simulink model "servoDirection"  (R2019a)
settings: Solver=VariableStepAuto  StartTime=0.0  StopTime=10.0  RelTol=1e-3
undefined symbols (not defined in the file or in its folder): DiscIntNeverNeededParam
libraries: embdlinuxlib x2, raspberrypilib x1
settings Model: Creator=wojna  LastModifiedBy=wojna

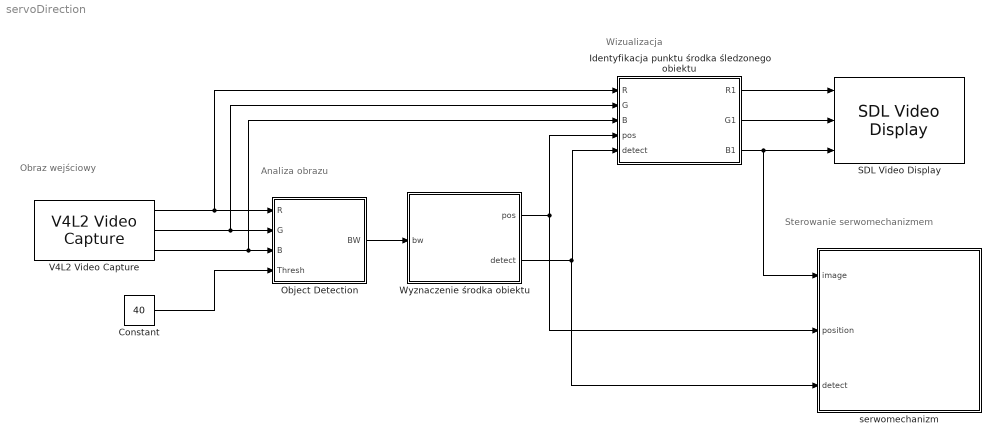
== system servoDirection ==
  note: Obraz wejściowy
  note: Sterowanie serwomechanizmem
  note: Wizualizacja
  note: Analiza obrazu
  Constant : Constant  Value=40
  Identyfikacja punktu środka śledzonego obiektu : MATLAB Function  TreatAsAtomicUnit=on
  Object Detection : Subsystem
  SDL Video Display : embdlinuxlib/SDL Video Display  pixelFormat=RGB  pixelOrder=Planar  rowMajor=on  blockPlatform=Raspberry Pi
      settings: SourceProductName=Simulink Coder Support Package for BeagleBone Blue Hardware  SourceProductBaseCode=SC_BEAGLEBONE_BLUE
  V4L2 Video Capture : embdlinuxlib/V4L2 Video Capture  m_devName='/dev/video0'  roi=[0, 0, 640, 480]  imSizeSelection=160x120  imSize=[640, 480]  pixelFormat=RGB  pixelOrder=Planar  sampleTime=0.05  simOutput=Colorbars  blockPlatform=Raspberry Pi
      settings: SourceProductName=Simulink Coder Support Package for BeagleBone Blue Hardware  SourceProductBaseCode=SC_BEAGLEBONE_BLUE
  Wyznaczenie środka obiektu : MATLAB Function  TreatAsAtomicUnit=on
  serwomechanizm : Subsystem
  wires:
  V4L2 Video Capture/1 -> Object Detection/1(R), Identyfikacja punktu środka śledzonego obiektu/1(R)
  V4L2 Video Capture/2 -> Object Detection/2(G), Identyfikacja punktu środka śledzonego obiektu/2(G)
  V4L2 Video Capture/3 -> Identyfikacja punktu środka śledzonego obiektu/3(B), Object Detection/3(B)
  Object Detection/1(BW) -> Wyznaczenie środka obiektu/1(bw)
  Wyznaczenie środka obiektu/1(pos) -> Identyfikacja punktu środka śledzonego obiektu/4(pos), serwomechanizm/2(position)
  Wyznaczenie środka obiektu/2(detect) -> serwomechanizm/3(detect), Identyfikacja punktu środka śledzonego obiektu/5(detect)
  Identyfikacja punktu środka śledzonego obiektu/1(R1) -> SDL Video Display/1
  Identyfikacja punktu środka śledzonego obiektu/2(G1) -> SDL Video Display/2
  Identyfikacja punktu środka śledzonego obiektu/3(B1) -> serwomechanizm/1(image), SDL Video Display/3
  Constant/1 -> Object Detection/4(Thresh)

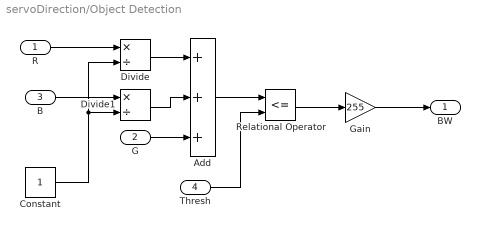
== system servoDirection/Object Detection ==
  R : Inport
  G : Inport  Port=2
  B : Inport  Port=3
  Thresh : Inport  Port=4
  Add : Sum  Inputs=+++
  Constant : Constant
  Divide : Product  Inputs=*/
  Divide1 : Product  Inputs=*/
  Gain : Gain  Gain=255
  Relational Operator : RelationalOperator  Operator=<=  OutDataTypeStr=boolean  RndMeth=Simplest
  BW : Outport
  wires:
  Thresh/1 -> Relational Operator/2
  Constant/1 -> Divide1/2, Divide/2
  Gain/1 -> BW/1
  Add/1 -> Relational Operator/1
  Divide1/1 -> Add/2
  Relational Operator/1 -> Gain/1
  Divide/1 -> Add/1
  R/1 -> Divide/1
  B/1 -> Divide1/1
  G/1 -> Add/3

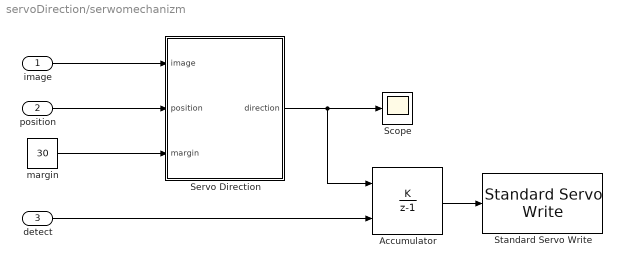
== system servoDirection/serwomechanizm ==
  image : Inport
  position : Inport  Port=2
  detect : Inport  Port=3
  Accumulator : DiscreteIntegrator  IntegratorMethod=Accumulation: Forward Euler  ExternalReset=falling  SampleTime=-1  LimitOutput=on  ICPrevOutput=DiscIntNeverNeededParam  ICPrevScaledInput=DiscIntNeverNeededParam
  Scope : Scope
  "Servo Direction " : Subsystem
  Standard Servo Write : raspberrypilib/Standard Servo Write  board=Pi 3 Model B  Pin_=18  MinPulseDuration=1000e-6  MaxPulseDuration=2000e-6  blockPlatform=Raspberry Pi
      settings: SourceProductName=Simulink Support Package for Raspberry Pi Hardware  SourceProductBaseCode=RASPPI
  margin : Constant  Value=30
  wires:
  "Servo Direction "/1("direction ") -> Accumulator/1, Scope/1
  detect/1 -> Accumulator/2
  Accumulator/1 -> Standard Servo Write/1
  margin/1 -> "Servo Direction "/3("margin ")
  position/1 -> "Servo Direction "/2(position)
  image/1 -> "Servo Direction "/1(image)

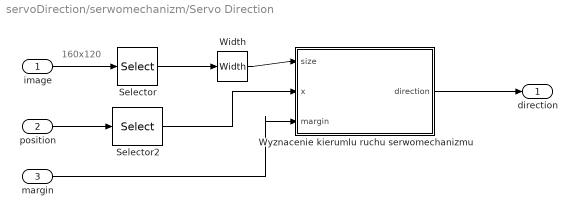
== system servoDirection/serwomechanizm/Servo Direction  ==
  note: 160x120
  image : Inport
  position : Inport  Port=2
  "margin " : Inport  Port=3
  Selector : Selector  NumberOfDimensions=2  InputPortWidth=160  IndexOptions=Select all,Select all  Indices=1,1  OutputSizes=160,1
  Selector2 : Selector  InputPortWidth=2  IndexOptions=Index vector (dialog)  Indices=[1]  OutputSizes=1
  Width : Width
  Wyznacenie kierumlu ruchu serwomechanizmu : MATLAB Function  TreatAsAtomicUnit=on
  "direction " : Outport
  wires:
  position/1 -> Selector2/1
  Wyznacenie kierumlu ruchu serwomechanizmu/1(direction) -> "direction "/1
  Selector2/1 -> Wyznacenie kierumlu ruchu serwomechanizmu/2(x)
  Width/1 -> Wyznacenie kierumlu ruchu serwomechanizmu/1(size)
  Selector/1 -> Width/1
  image/1 -> Selector/1
  "margin "/1 -> Wyznacenie kierumlu ruchu serwomechanizmu/3(margin)

== matlab function servoDirection/Wyznaczenie środka obiektu ==
  data: bw input; pos output; detect output
function [pos, detect] = FindCentroid(bw)

[r,c]=find(bw);
if isempty(r)
    pos = [-1 -1];
    detect = false;
else
    pos = [mean(r), mean(c)];
    detect = true;
end

== matlab function servoDirection/Identyfikacja punktu środka śledzonego obiektu ==
  data: R input; R1 output; G input; B input; pos input; detect input; G1 output; B1 output
function [R1,G1,B1] = MarkImage(R,G,B, pos, detect)
R1 = R; G1 = G; B1 = B;
if detect
    R1(pos(1)-3:pos(1)+3, pos(2)-3:pos(2)+3) = 255;
    G1(pos(1)-3:pos(1)+3, pos(2)-3:pos(2)+3) = 0; 
    B1(pos(1)-3:pos(1)+3, pos(2)-3:pos(2)+3) = 0;
end

== matlab function servoDirection/serwomechanizm/Servo Direction /Wyznacenie kierumlu ruchu serwomechanizmu ==
  data: size input; direction output; x input; margin input
function direction = servoDirection(size, x, margin)

center = size / 2;
if x == -1
    direction = 0;
elseif x >= center + margin
    direction = 1;
elseif x <= center - margin
    direction = -1;
else 
    direction = 0;
end
